simulink model "Project1_Part1"  (R2023b)
settings: Solver=ode1  StartTime=0.0  StopTime=25  FixedStep=0.1  RelTol=1e-3
values from neighbouring files (symbols this model uses):
  A_var = A(i)    [Project1_Part2_matlab.m]    (also in init.m = 0; plotting_loop.m = 100)
  b_var = 0    [init.m]    (also in plotting_loop.m = b(k))
  freq = 1    [init.m]    (also in plotting_loop.m = freq_var(f))
  J_var = 0    [init.m]    (also in plotting_loop.m = J(j))
  switch_value = 0    [init.m]    (also in plotting_loop.m = sin_var(o))
  w_0_var = 0    [init.m]    (also in plotting_loop.m = w_0(i))
settings Model: Creator=saman  LastModifiedBy=xavie

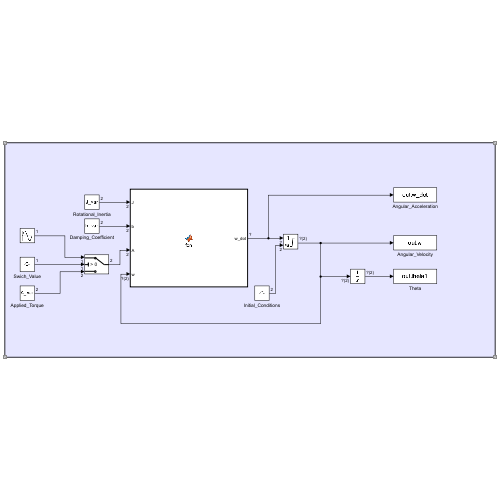
[thumbnail: Simulink's stored preview of the top-level diagram]
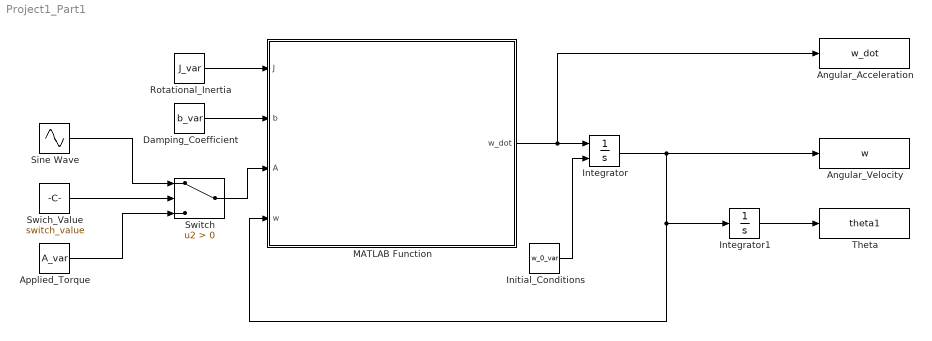
== system Project1_Part1 ==
  Angular_Acceleration : ToWorkspace  VariableName=w_dot  SaveFormat=Timeseries  SampleTime=-1
  Angular_Velocity : ToWorkspace  VariableName=w  SaveFormat=Timeseries  SampleTime=-1
  Applied_Torque : Constant  Value=A_var
  Damping_Coefficient : Constant  Value=b_var
  Initial_Conditions : Constant  Value=w_0_var
  Integrator : Integrator  InitialConditionSource=external  LimitOutput=on  UpperSaturationLimit=10000  LowerSaturationLimit=0
  Integrator1 : Integrator
  MATLAB Function : MATLAB Function  TreatAsAtomicUnit=on
  Rotational_Inertia : Constant  Value=J_var
  Sine Wave : Sin  Amplitude=A_var  Frequency=freq  SampleTime=0
  Swich_Value : Constant  Value=switch_value
  Switch : Switch  Criteria=u2 > Threshold  SaturateOnIntegerOverflow=off  InputSameDT=off
  Theta : ToWorkspace  VariableName=theta1  SaveFormat=Timeseries  SampleTime=-1
  wires:
  Rotational_Inertia/1 -> MATLAB Function/1(J)
  Damping_Coefficient/1 -> MATLAB Function/2(b)
  MATLAB Function/1(w_dot) -> Angular_Acceleration/1, Integrator/1
  Initial_Conditions/1 -> Integrator/2
  Integrator/1 -> Angular_Velocity/1, Integrator1/1, MATLAB Function/4(w)
  Integrator1/1 -> Theta/1
  Applied_Torque/1 -> Switch/3
  Swich_Value/1 -> Switch/2
  Sine Wave/1 -> Switch/1
  Switch/1 -> MATLAB Function/3(A)

== matlab function Project1_Part1/MATLAB Function ==
  data: J input; w_dot output; b input; A input; w input
function w_dot = fcn(J, b, A,w)
tau_damped = b * w;
w_dot = (1/J)*(A-tau_damped);
end
